simulink model "PSK"  (R2022b)
settings: Solver=VariableStepAuto  StartTime=0.0  StopTime=stop_time  RelTol=1e-3
libraries: commdigbbndpm3 x2, commchan3 x1, commsink2 x1, commrandsrc3 x1
settings Model: Creator=g  LastModifiedBy=g

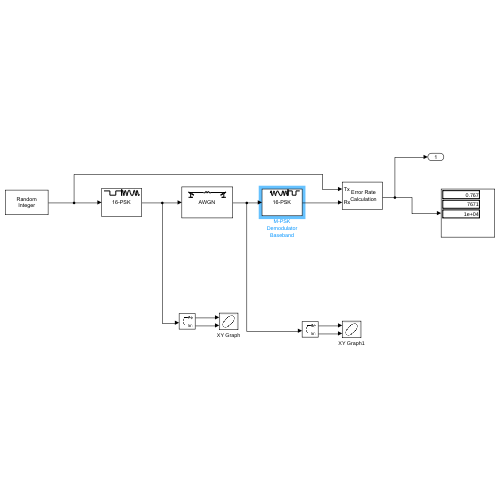
[thumbnail: Simulink's stored preview of the top-level diagram]
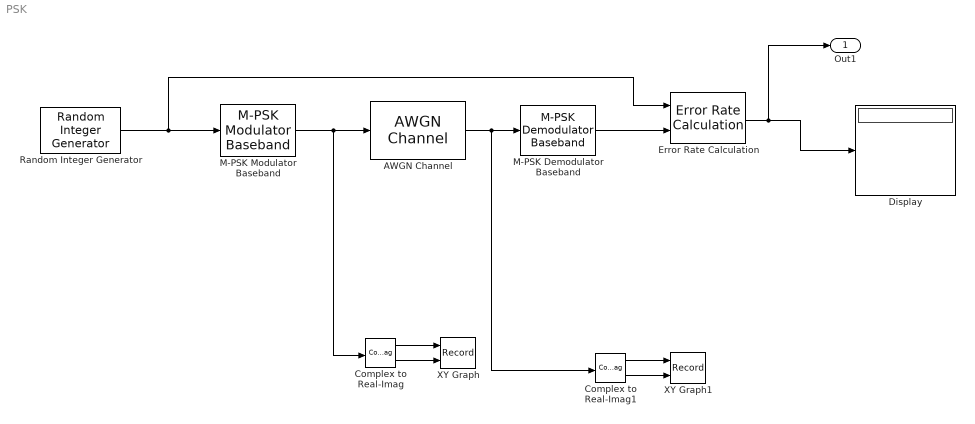
== system PSK ==
  AWGN Channel : commchan3/AWGN Channel  InputProcessing=Columns as channels (frame based)  seed=67  noiseMode="Signal to noise ratio  (Eb/No)"  EbNodB=Eb_No_db  EsNodB=10  SNRdB=10  bitsPerSym=2  Ps=1  Tsym=0.2  variance=1
  Complex to Real-Imag : ComplexToRealImag
  Complex to Real-Imag1 : ComplexToRealImag
  Display : Display
  Error Rate Calculation : commsink2/Error Rate Calculation  N=0  st_delay=0  cp_mode=Entire frame  subframe=[]  PMode=Port  WsName=ErrorVec  RsMode2=off  stop=off  numErr=100  maxBits=1e6
  M-PSK Demodulator Baseband : commdigbbndpm3/M-PSK Demodulator Baseband  M=m_ary  OutType=Integer  DecType=Hard decision  VarSource=Dialog  Variance=1  Dec=Gray  Mapping=[0:7]  Ph=phaseOffset  outDtype1=Inherit via internal rule  outDtype2=Inherit via internal rule  derotateFactorWordLen=16  derotateFactorDataTypeStr=Inherit: Same word length as input  derotateFactorLastDataTypeStr=Inherit: Same word length as input
  M-PSK Modulator Baseband : commdigbbndpm3/M-PSK Modulator Baseband  M=m_ary  InType=Integer  Enc=Gray  Mapping=[0:7]  Ph=phaseOffset  outDtype=double  outWordLen=16  outUDDataType=sfix(16)  outFracLenMode=Best precision  outFracLen=15  outDataTypeStr=double  outLastDataTypeStr=double
  Random Integer Generator : commrandsrc3/Random Integer Generator  SetSize=m_ary  SeedSource=Auto  Seed=0  SampleTime=0.1  SamplesPerFrame=1  OutputDataType=double  SimulateUsing=Interpreted execution
  XY Graph : Record  FileSettingsInternal="{\"entries\":[{\"content\":{\"excelSettings\":{\"content\":{},\"type\":\"Streamout.ExcelSettings\"}},\"type\":\"Streamout.FileSettingStorage\",\"uuid\":\"faa23d01-f14c-4597-a616-2f0d9fd09a3a\"}],\"packageUris\":[\"http://schema.mathworks.com/mf0/streamout_blocks/R2020a\"],\"version\":\"1.0\"}"  Layout=[1 1]  SignalsInternal="{\"entries\":[{\"content\":{\"signals\":[{\"content\":{\"blockPath\":[\"PSK/XY Graph\"],\"channel\":[],\"dimensions\":[1,1],\"domain\":\"PSK/XY Graph\",\"lineColor\":\"#a2142f\",\"plots\":[1],\"port\":1,\"sid\":[\"\"],\"signalID\":93845,\"signalName\":\"Complex to\\nReal-Imag:1\"},\"type\":\"RecordBlkView.Signal\",\"uuid\":\"81a16c8e-8c26-48b4-8cb0-c14766d13621\"},{\"content\":{\"blockPath\":[\"PSK/XY Graph\"],\"channel\":[],\"dimensions\":[1,1],\"domain\":\"PSK/XY Graph\",\"lineColor\":\"#139fff\",\"plots\":[1],\"port\":2,\"sid\":[\"\"],\"signalID\":93849,\"signalName\":\"Complex to\\nReal-Imag:2\"},\"type\":\"RecordBlkView.Signal\",\"uuid\":\"0ea63d54-6205-4d44-9855-ab99f68ff290\"}]},\"type\":\"RecordBlkView.InputSignals\",\"uuid\":\"d7048a46-c1a8-44e0-83dd-b4ac663b4a4c\"}],\"packageUris\":[\"http://schema.mathworks.com/mf0/streamout_blocks/R2020a\"],\"version\":\"1.0\"}"  VisualizationBindings="{\"xyplotplugin\":{\"info\":[{\"series\":[{\"bindingParametersList\":[{\"parameter\":\"X-Axis\",\"signalID\":93845,\"signalName\":\"Complex to\\nReal-Imag:1\"},{\"parameter\":\"Y-Axis\",\"signalID\":93849,\"signalName\":\"Complex to\\nReal-Imag:2\"}],\"seriesID\":24572}],\"subplotID\":1}]}}"  CompatibilityTag=XY
  XY Graph1 : Record  FileSettingsInternal="{\"entries\":[{\"content\":{\"excelSettings\":{\"content\":{},\"type\":\"Streamout.ExcelSettings\"}},\"type\":\"Streamout.FileSettingStorage\",\"uuid\":\"36fdd813-2855-48c1-92e1-6f3eabdb8516\"}],\"packageUris\":[\"http://schema.mathworks.com/mf0/streamout_blocks/R2020a\"],\"version\":\"1.0\"}"  Layout=[1 1]  SignalsInternal="{\"entries\":[{\"content\":{\"signals\":[{\"content\":{\"blockPath\":[\"PSK/XY Graph1\"],\"channel\":[],\"dimensions\":[1,1],\"domain\":\"PSK/XY Graph1\",\"lineColor\":\"#a2142f\",\"plots\":[1],\"port\":1,\"sid\":[\"\"],\"signalID\":93853,\"signalName\":\"Complex to\\nReal-Imag1:1\"},\"type\":\"RecordBlkView.Signal\",\"uuid\":\"e7b366e4-3a82-4912-8bb3-aa1241130bf1\"},{\"content\":{\"blockPath\":[\"PSK/XY Graph1\"],\"channel\":[],\"dimensions\":[1,1],\"domain\":\"PSK/XY Graph1\",\"lineColor\":\"#139fff\",\"plots\":[1],\"port\":2,\"sid\":[\"\"],\"signalID\":93857,\"signalName\":\"Complex to\\nReal-Imag1:2\"},\"type\":\"RecordBlkView.Signal\",\"uuid\":\"631b6310-1106-4040-8d99-2b8b61d56b09\"}]},\"type\":\"RecordBlkView.InputSignals\",\"uuid\":\"35ecc172-04d0-4ae9-99a3-7cea8cc990a1\"}],\"packageUris\":[\"http://schema.mathworks.com/mf0/streamout_blocks/R2020a\"],\"version\":\"1.0\"}"  VisualizationBindings="{\"xyplotplugin\":{\"info\":[{\"series\":[{\"bindingParametersList\":[{\"parameter\":\"X-Axis\",\"signalID\":93853,\"signalName\":\"Complex to\\nReal-Imag1:1\"},{\"parameter\":\"Y-Axis\",\"signalID\":93857,\"signalName\":\"Complex to\\nReal-Imag1:2\"}],\"seriesID\":16207}],\"subplotID\":1}]}}"  CompatibilityTag=XY
  Out1 : Outport
  wires:
  Random Integer Generator/1 -> M-PSK Modulator Baseband/1, Error Rate Calculation/1
  M-PSK Modulator Baseband/1 -> Complex to Real-Imag/1, AWGN Channel/1
  AWGN Channel/1 -> M-PSK Demodulator Baseband/1, Complex to Real-Imag1/1
  M-PSK Demodulator Baseband/1 -> Error Rate Calculation/2
  Error Rate Calculation/1 -> Out1/1, Display/1
  Complex to Real-Imag/1 -> XY Graph/1
  Complex to Real-Imag/2 -> XY Graph/2
  Complex to Real-Imag1/1 -> XY Graph1/1
  Complex to Real-Imag1/2 -> XY Graph1/2
